simulink library "acc"  (R2021b)
settings: Solver=VariableStepAuto  StartTime=0.0  StopTime=10.0  RelTol=1e-3
undefined symbols (not defined in the file or in its folder): AACC_CondensorFanReq_X_enum, AACC_EWP1CCUReq_X_C, AACC_EWP1EDUReq_X_C, AACC_EWP1HVBReq_X_C, AACC_EWP2CCUReq_X_C, AACC_EWP2EDUReq_X_C, AACC_EWP2HVBReq_X_C, AACC_FWV1CCUReq_X_C, AACC_FWV1EDUReq_X_C, AACC_FWV1HVBReq_X_C, AACC_FWV2CCUReq_X_C, AACC_FWV2EDUReq_X_C, AACC_FWV2HVBReq_X_C, AACC_TWVCCUReq_X_C, AACC_TWVEDUReq_X_C, AACC_TWVHVBReq_X_C, ENUM_ACCMODE_CHARGING, ENUM_ACCMODE_COOLING, ENUM_ACCMODE_OFF, ENUM_ACCMODE_SERVICE, ENUM_ACREQ_COOLING, ENUM_ACREQ_NOREQUEST, ENUM_CHILLERINITREQ_NONE, ENUM_CHILLERINITREQ_START, ENUM_CHILLERINITREQ_WAITING, ENUM_CHILLERINITSTA_FINISH, ENUM_CHILLERINITSTA_INPROCESS, ENUM_COOLFANREQ_HI, ENUM_COOLFANREQ_LOW, ENUM_COOLFANREQ_OFF, ENUM_EACENDEM_SHUTDOWN, ENUM_EACENDEM_START, ENUM_EACENSTA_RUN, ENUM_EBSBRKSW_PRESSED, ENUM_EBSBRKSW_RELEASED, ENUM_EHPSENDEM_SHUTDOWN, ENUM_EHPSENDEM_START, ENUM_EPBSTARAW_SET, ENUM_GEARACTUALPOSN_N, ENUM_GEARACTUALPOSN_P, ENUM_LVBATTSTA_FAIL, ENUM_LVBATTSTA_NORMAL, ENUM_PMMMODE_CHARGE, ENUM_PMMMODE_DRIVE, ENUM_PMMMODE_LVBATCHRG, ENUM_PMMMODE_POWERUP, ENUM_POWERSTA_OFF, ENUM_POWERSTA_ON, ENUM_POWERSTA_READY, ENUM_POWERSTA_STANDBY, ENUM_PUSTATE_COMPLETED, ENUM_THCMSYS_INACTIVE, FALSE, KACC_CACEnableFailTime_s, KACC_CCUFanHighOffTemp_C, KACC_CCUFanHighOnTemp_C, KACC_CCUFanLowOffTemp_C, KACC_CCUFanLowOnTemp_C, KACC_ChillerInitTime_s, KACC_ChillerStartTime_s ... (+77)
libraries: hcu_lib x10, simulink x1
(part 1 of 2)
settings Model: Creator=13615  LastModifiedBy=zack
settings SolverCC: AlgebraicLoopSolver=TrustRegion
settings DataIOCC: SaveFormat=Array  SignalLoggingSaveFormat=ModelDataLogs  ReturnWorkspaceOutputs=off
settings OptimizationCC: BlockReduction=off  BooleanDataType=off
settings DebuggingCC: SaveWithParameterizedLinksMsg=none  UnderspecifiedInitializationDetection=Classic  MergeDetectMultiDrivingBlocksExec=none  SignalResolutionControl=TryResolveAllWithWarning  SFMachineParentedDataDiag=warning  ArithmeticOperatorsInVariantConditions=warning
settings HardwareCC: TargetUnknown=on
settings ModelReferenceCC: PropagateSignalLabelsOutOfModel=off
settings SFSimCC: CustomCodeUndefinedFunction=UseInterfaceOnly
settings ConfigComp: CovMetricSettings=dw  CovSaveCumulativeToWorkspaceVar=on  CovSaveSingleToWorkspaceVar=on

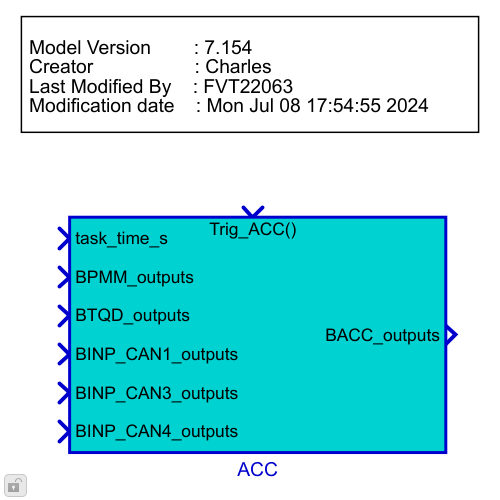
[thumbnail: Simulink's stored preview of the top-level diagram]
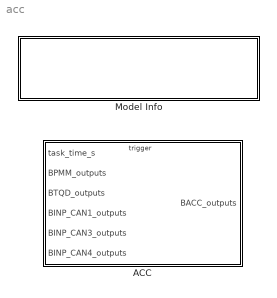
== system acc ==
  ACC : Subsystem  TreatAsAtomicUnit=on
      settings: RTWSystemCode=Nonreusable function  RTWFcnNameOpts=Use subsystem name  RTWFileNameOpts=Use subsystem name
  Model Info : Subsystem  LoadFcn=slcm LoadBlock;  InitFcn=slcm('UpdateAllCMBlocksInThisModelInit')  mask(CMBlock){InitialSaveTempField=, InitialBlockCM=None, BlockCM=None, Frame=on, SaveTempField=, DisplayStringWithTags=|, MaskDisplayString=Model Version        : 7.186\nCreator                   : Charles\nLast Modified By    : zack\nModification date    : Thu Aug 22 11:54:03 2024, HorizontalTextAlignment=Left, LeftAlignmentValue=0.02, SourceBlockDiagram=acc, TagMaxNumber=20, CMTag1=, CMTag2=, CMTag3=, CMTag4=, CMTag5=, CMTag6=, CMTag7=, CMTag8=, CMTag9=, CMTag10=, CMTag11=, CMTag12=, CMTag13=, CMTag14=, CMTag15=, CMTag16=, CMTag17=, CMTag18=, CMTag19=, CMTag20=}
      mask DisplayStringWithTags=|
      | Model Version        : %<ModelVersion>
      | Creator                   : Charles
      | Last Modified By    : %<LastModifiedBy>
      | Modification date    : %<LastModificationDate>
      mask help: This block allows revision control information to be displayed within the model.
      settings: CopyFcn=slcm CopyBlock;  DeleteFcn=slcm Cancel;  PostSaveFcn=slcm('UpdateAllCMBlocksInThisModel')  NameChangeFcn=slcm Rename;  OpenFcn=slcm
      mask Display: text(str2num(LeftAlignmentValue), 0.5, MaskDisplayString, 'HorizontalAlignment', HorizontalTextAlignment)

== system acc/ACC ==
  task_time_s : Inport
  BPMM_outputs : Inport  Port=2  OutDataTypeStr=Bus: BPMM_outputs
  BTQD_outputs : Inport  Port=3  OutDataTypeStr=Bus: BTQD_outputs
  BINP_CAN1_outputs : Inport  Port=4  OutDataTypeStr=Bus: BINP_CAN1_outputs
  BINP_CAN3_outputs : Inport  Port=5  OutDataTypeStr=Bus: BINP_CAN3_outputs
  BINP_CAN4_outputs : Inport  Port=6  OutDataTypeStr=Bus: BINP_CAN4_outputs
  Trig_ACC : TriggerPort  TriggerType=function-call  VariantControl=(inherit)
  ACC : Subsystem
  ACC1 : Subsystem  Commented=on  AncestorBlock=acc/ACC/ACC
  Bus Creator : BusCreator  Inputs=8  OutDataTypeStr=Bus: BACC_outputs  NonVirtualBus=on
  Bus Selector1 : BusSelector  OutputSignals=VINP_LVBattDet12V_V,VINP_HVBPwrAvailDchrg_kW,VINP_RrMCUDCBusVolt_V,VINP_RrMCUDCBusCurr_A
  Bus Selector2 : BusSelector  OutputSignals=VPMM_HVPwrSta_flg,VPMM_LVPwrSta_flg,VPMM_PowerSta_enum
  Bus Selector3 : BusSelector  OutputSignals=VINP_FASpeed_kph,VINP_EBSBrakeSw_enum,VINP_EACEnSta_enum,VINP_EPBParkingBrakeSta_enum
  Bus Selector4 : BusSelector  OutputSignals=VTQD_GearActualPosn_enum
  Bus Selector5 : BusSelector  OutputSignals=VINP_Z24CHAAirPressureFC2Sta_KPa,VINP_Z24CHAAirPressurePC3Sta_KPa,VINP_Z24CHAAirPressureRC1Sta_KPa
  Model Info : simulink/Model-Wide Utilities/Model Info  Frame=on  DisplayStringWithTags=|  HorizontalTextAlignment=Center  LeftAlignmentValue=0.5
      | $Id: ACC.mdl 2018-05-29 Lon $
      | Modified By %<ModifiedBy>
      | Modified Date : %<ModifiedDate>
  BACC_outputs : Outport  OutDataTypeStr=Bus: BACC_outputs  VectorParamsAs1DForOutWhenUnconnected=off
  wires:
  BPMM_outputs/1 -> Bus Selector2/1
  Bus Creator/1 -> BACC_outputs/1  "BACC_outputs"
  BINP_CAN3_outputs/1 -> Bus Selector1/1
  Bus Selector1/1 -> ACC/5(VINP_LVBattDet12V_V)  "<VINP_LVBattDet12V_V>"
  task_time_s/1 -> ACC/1(task_time_s)  "task_time_s"
  Bus Selector1/2 -> ACC/6(VINP_HVBPwrAvailDchrg_kW)  "<VINP_HVBPwrAvailDchrg_kW>"
  Bus Selector1/3 -> ACC/7(VINP_RrMCUDCBusVolt_V)  "<VINP_RrMCUDCBusVolt_V>"
  Bus Selector1/4 -> ACC/8(VINP_RrMCUDCBusCurr_A)  "<VINP_RrMCUDCBusCurr_A>"
  ACC/3(VACC_VehHVPwrAvail4THCM_W) -> Bus Creator/3
  ACC/1(VACC_HVTHCMSysAvail_enum) -> Bus Creator/1
  ACC/2(VACC_LVBattVoltSta_enum) -> Bus Creator/2
  Bus Selector2/1 -> ACC/2(VPMM_HVPwrSta_flg)  "<VPMM_HVPwrSta_flg>"
  Bus Selector2/2 -> ACC/3(VPMM_LVPwrSta_flg)  "<VPMM_LVPwrSta_flg>"
  ACC/4(VACC_EHPSEnDem_enum) -> Bus Creator/4
  ACC/5(VACC_CACPresWarnSta_flg) -> Bus Creator/5
  ACC/6(VACC_CACTempWarnSta_flg) -> Bus Creator/6
  ACC/7(VACC_EACEnDem_enum) -> Bus Creator/7
  ACC/8(VACC_EACPreSelfChkSta_flg) -> Bus Creator/8
  BINP_CAN1_outputs/1 -> Bus Selector3/1
  Bus Selector3/3 -> ACC/12(VINP_EACEnSta_enum)  "<VINP_EACEnSta_enum>"
  Bus Selector3/1 -> ACC/10(VINP_FASpeed_kph)  "<VINP_FASpeed_kph>"
  Bus Selector3/2 -> ACC/11(VINP_EBSBrakeSW_enum)  "<VINP_EBSBrakeSw_enum>"
  Bus Selector2/3 -> ACC/4(VPMM_PowerSta_enum)  "<VPMM_PowerSta_enum>"
  BTQD_outputs/1 -> Bus Selector4/1
  Bus Selector4/1 -> ACC/9(VTQD_GearActualPosn_enum)  "<VTQD_GearActualPosn_enum>"
  BINP_CAN4_outputs/1 -> Bus Selector5/1
  Bus Selector5/1 -> ACC/14(VINP_Z24CHAAirPressureFC2Sta_kPa)  "<VINP_Z24CHAAirPressureFC2Sta_KPa>"
  Bus Selector5/2 -> ACC/15(VINP_Z24CHAAirPressurePC3Sta_kPa)  "<VINP_Z24CHAAirPressurePC3Sta_KPa>"
  Bus Selector5/3 -> ACC/16(VINP_Z24CHAAirPressureRC1Sta_kPa)  "<VINP_Z24CHAAirPressureRC1Sta_KPa>"
  Bus Selector3/4 -> ACC/13(VINP_EPBParkingBrakeSta_enum)  "<VINP_EPBParkingBrakeSta_enum>"

== system acc/Model Info ==
  EmptySubsystem : Subsystem

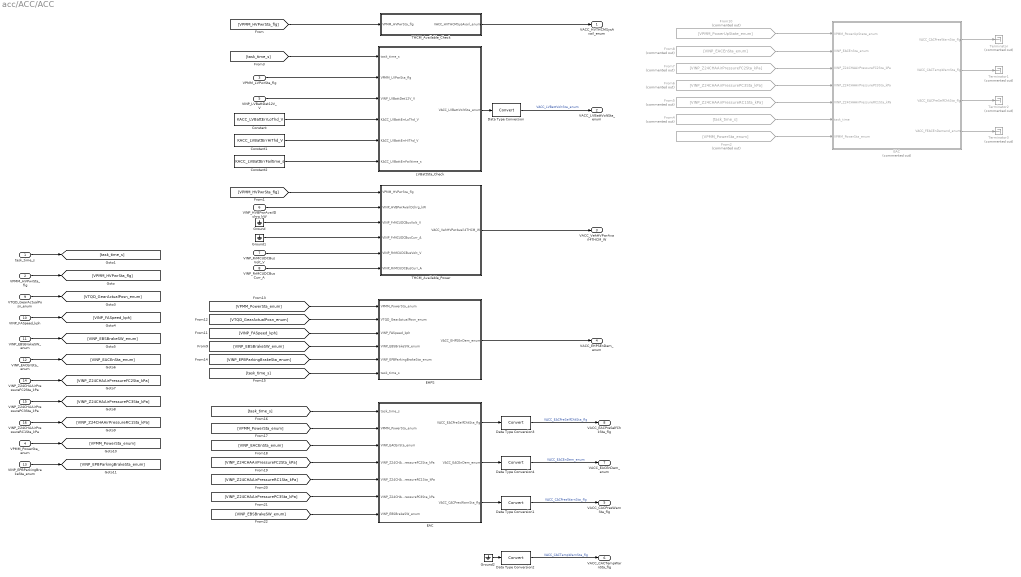
== system acc/ACC/ACC ==
  task_time_s : Inport
  VPMM_HVPwrSta_flg : Inport  Port=2
  VPMM_LVPwrSta_flg : Inport  Port=3
  VPMM_PowerSta_enum : Inport  Port=4
  VINP_LVBattDet12V_V : Inport  Port=5
  VINP_HVBPwrAvailDchrg_kW : Inport  Port=6
  VINP_RrMCUDCBusVolt_V : Inport  Port=7
  VINP_RrMCUDCBusCurr_A : Inport  Port=8
  VTQD_GearActualPosn_enum : Inport  Port=9
  VINP_FASpeed_kph : Inport  Port=10
  VINP_EBSBrakeSW_enum : Inport  Port=11
  VINP_EACEnSta_enum : Inport  Port=12
  VINP_EPBParkingBrakeSta_enum : Inport  Port=13
  VINP_Z24CHAAirPressureFC2Sta_kPa : Inport  Port=14
  VINP_Z24CHAAirPressurePC3Sta_kPa : Inport  Port=15
  VINP_Z24CHAAirPressureRC1Sta_kPa : Inport  Port=16
  Constant : Constant  Value=KACC_LVBattErrLoThd_V
  Constant1 : Constant  Value=KACC_LVBattErrHiThd_V
  Constant2 : Constant  Value=KACC_LVBattErrFailtime_s
  Data Type Conversion{,1..4} (5 alike) : DataTypeConversion
  EAC : Stateflow chart  Commented=on  TreatAsAtomicUnit=on
  "EAC " : Subsystem
  EHPS : Subsystem
  From10 : From  Commented=on  GotoTag=VPMM_PowerUpState_enum
  From2 : From  Commented=on  GotoTag=VPMM_PowerSta_enum
  From4 : From  Commented=on  GotoTag=task_time_s
  From5 : From  Commented=on  GotoTag=VINP_Z24CHAAirPressureRC1Sta_kPa
  From6 : From  Commented=on  GotoTag=VINP_Z24CHAAirPressurePC3Sta_kPa
  From7 : From  Commented=on  GotoTag=VINP_Z24CHAAirPressureFC2Sta_kPa
  From8 : From  Commented=on  GotoTag=VINP_EACEnSta_enum
  Ground : Ground
  Ground1 : Ground
  Ground2 : Ground
  LVBattSta_Check : Stateflow chart  TreatAsAtomicUnit=on
  THCM_Available_Check : Subsystem
  THCM_Available_Power : Subsystem
  Terminator{,1..3} (4 alike) : Terminator  Commented=on
  VACC_HVTHCMSysAvail_enum : Outport
  VACC_LVBattVoltSta_enum : Outport  Port=2
  VACC_VehHVPwrAvail4THCM_W : Outport  Port=3
  VACC_EHPSEnDem_enum : Outport  Port=4
  VACC_CACPresWarnSta_flg : Outport  Port=5
  VACC_CACTempWarnSta_flg : Outport  Port=6
  VACC_EACEnDem_enum : Outport  Port=7
  VACC_EACPreSelfChkSta_flg : Outport  Port=8
  wires:
  VINP_LVBattDet12V_V/1 -> LVBattSta_Check/3(VINP_LVBattDet12V_V)
  Constant/1 -> LVBattSta_Check/4(KACC_LVBattErrLoThd_V)
  Constant1/1 -> LVBattSta_Check/5(KACC_LVBattErrHiThd_V)
  Constant2/1 -> LVBattSta_Check/6(KACC_LVBattErrFailtime_s)
  LVBattSta_Check/1(VACC_LVBattVoltSta_enum) -> Data Type Conversion/1
  task_time_s/1 -> [task_time_s]
  VPMM_HVPwrSta_flg/1 -> [VPMM_HVPwrSta_flg]
  Data Type Conversion/1 -> VACC_LVBattVoltSta_enum/1  "VACC_LVBattVoltSta_enum"
  VPMM_LVPwrSta_flg/1 -> LVBattSta_Check/2(VPMM_LVPwrSta_flg)
  [VPMM_HVPwrSta_flg] -> THCM_Available_Check/1(VPMM_HVPwrSta_flg)
  THCM_Available_Check/1(VACC_HVTHCMSysAvail_enum) -> VACC_HVTHCMSysAvail_enum/1
  [VPMM_HVPwrSta_flg] -> THCM_Available_Power/1(VPMM_HVPwrSta_flg)
  THCM_Available_Power/1(VACC_VehHVPwrAvail4THCM_W) -> VACC_VehHVPwrAvail4THCM_W/1
  Ground/1 -> THCM_Available_Power/3(VINP_FrMCUDCBusVolt_V)
  Ground1/1 -> THCM_Available_Power/4(VINP_FrMCUDCBusCurr_A)
  VINP_RrMCUDCBusVolt_V/1 -> THCM_Available_Power/5(VINP_RrMCUDCBusVolt_V)
  VINP_RrMCUDCBusCurr_A/1 -> THCM_Available_Power/6(VINP_RrMCUDCBusCurr_A)
  VINP_HVBPwrAvailDchrg_kW/1 -> THCM_Available_Power/2(VINP_HVBPwrAvailDchrg_kW)
  From10/1 -> EAC/1(VPMM_PowerUpState_enum)
  From2/1 -> EAC/7(VPMM_PowerSta_enum)
  [task_time_s] -> LVBattSta_Check/1(task_time_s)
  From4/1 -> EAC/6(task_time)
  From8/1 -> EAC/2(VINP_EACEnSta_enum)
  From7/1 -> EAC/3(VINP_Z24CHAAirPressureFC2Sta_kPa)
  From6/1 -> EAC/4(VINP_Z24CHAAirPressurePC3Sta_kPa)
  From5/1 -> EAC/5(VINP_Z24CHAAirPressureRC1Sta_kPa)
  [VINP_EBSBrakeSW_enum] -> EHPS/4(VINP_EBSBrakeSW_enum)
  [VINP_FASpeed_kph] -> EHPS/3(VINP_FASpeed_kph)
  [VTQD_GearActualPosn_enum] -> EHPS/2(VTQD_GearActualPosn_enum)
  EHPS/1(VACC_EHPSEnDem_enum) -> VACC_EHPSEnDem_enum/1
  Data Type Conversion1/1 -> VACC_CACPresWarnSta_flg/1  "VACC_CACPresWarnSta_flg"
  Data Type Conversion2/1 -> VACC_CACTempWarnSta_flg/1  "VACC_CACTempWarnSta_flg"
  Data Type Conversion3/1 -> VACC_EACPreSelfChkSta_flg/1  "VACC_EACPreSelfChkSta_flg"
  Data Type Conversion4/1 -> VACC_EACEnDem_enum/1  "VACC_EACEnDem_enum"
  VTQD_GearActualPosn_enum/1 -> [VTQD_GearActualPosn_enum]
  VINP_FASpeed_kph/1 -> [VINP_FASpeed_kph]
  VINP_EBSBrakeSW_enum/1 -> [VINP_EBSBrakeSW_enum]
  VINP_EACEnSta_enum/1 -> [VINP_EACEnSta_enum]
  VINP_Z24CHAAirPressureFC2Sta_kPa/1 -> [VINP_Z24CHAAirPressureFC2Sta_kPa]
  VINP_Z24CHAAirPressurePC3Sta_kPa/1 -> [VINP_Z24CHAAirPressurePC3Sta_kPa]
  VINP_Z24CHAAirPressureRC1Sta_kPa/1 -> [VINP_Z24CHAAirPressureRC1Sta_kPa]
  VPMM_PowerSta_enum/1 -> [VPMM_PowerSta_enum]
  [VINP_EPBParkingBrakeSta_enum] -> EHPS/5(VINP_EPBParkingBrakeSta_enum)
  VINP_EPBParkingBrakeSta_enum/1 -> [VINP_EPBParkingBrakeSta_enum]
  [VPMM_PowerSta_enum] -> EHPS/1(VPMM_PowerSta_enum)
  [task_time_s] -> EHPS/6(task_time_s)
  EAC/1(VACC_CACPresWarnSta_flg) -> Terminator/1
  EAC/2(VACC_CACTempWarnSta_flg) -> Terminator1/1
  EAC/3(VACC_EACPreSelfChkSta_flg) -> Terminator2/1
  EAC/4(VACC_FEACEnDemand_enum) -> Terminator3/1
  [task_time_s] -> "EAC "/1(task_time_s)
  [VPMM_PowerSta_enum] -> "EAC "/2(VPMM_PowerSta_enum)
  [VINP_EACEnSta_enum] -> "EAC "/3(VINP_EACEnSta_enum)
  [VINP_Z24CHAAirPressureFC2Sta_kPa] -> "EAC "/4(VINP_Z24CHAAirPressureFC2Sta_kPa)
  [VINP_Z24CHAAirPressureRC1Sta_kPa] -> "EAC "/5(VINP_Z24CHAAirPressureRC1Sta_kPa)
  [VINP_Z24CHAAirPressurePC3Sta_kPa] -> "EAC "/6(VINP_Z24CHAAirPressurePC3Sta_kPa)
  [VINP_EBSBrakeSW_enum] -> "EAC "/7(VINP_EBSBrakeSW_enum)
  "EAC "/3(VACC_CACPresWarnSta_flg) -> Data Type Conversion1/1
  "EAC "/1(VACC_EACPreSelfChkSta_flg) -> Data Type Conversion3/1
  "EAC "/2(VACC_EACEnDem_enum) -> Data Type Conversion4/1
  Ground2/1 -> Data Type Conversion2/1

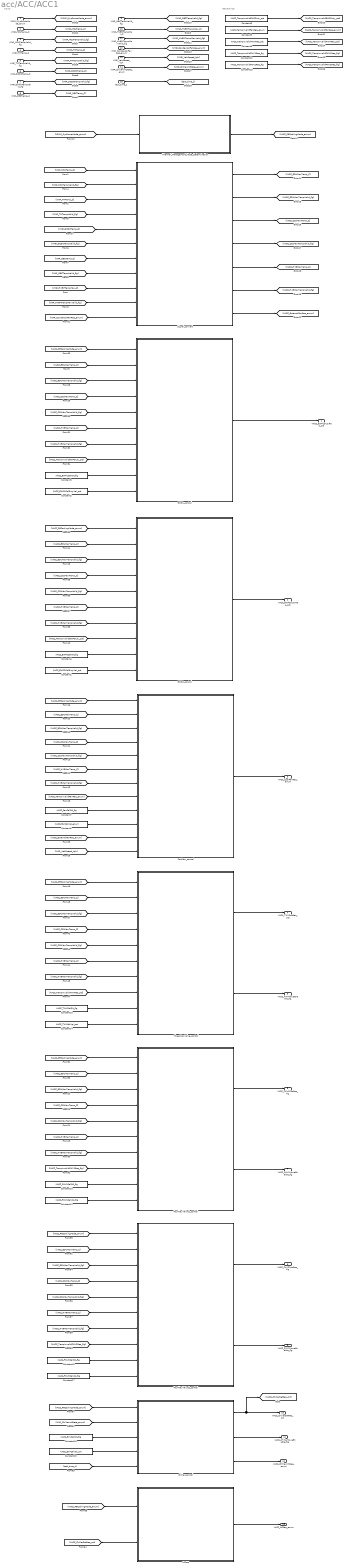
== system acc/ACC/ACC1 ==
  note: General Cal
  note: Inputs
  VPMM_SysPowerMode_enum : Inport
  VINP_MCUTemp_C : Inport  Port=2
  VINP_MCUTempValid_flg : Inport  Port=3
  VINP_TMTemp_C : Inport  Port=4
  VINP_TMTempValid_flg : Inport  Port=5
  VINP_DCDCTemp_C : Inport  Port=6
  VINP_DCDCTempValid_flg : Inport  Port=7
  VINP_OBCTemp_C : Inport  Port=8
  VINP_OBCTempValid_flg : Inport  Port=9
  VINP_HVBMTempMax_C : Inport  Port=10
  VINP_HVBMTempMaxValid_flg : Inport  Port=11
  VINP_CondensorFanReq_enum : Inport  Port=12
  VINP_VehSpeed_kph : Inport  Port=13
  VINP_ChillerInitState_enum : Inport  Port=14
  task_time_s : Inport  Port=15
  ACReq : Subsystem
  Chiller_control : Subsystem
  Constant1 : Constant  Value=KACC_EWP2CalDutyVal_pct
  Constant10 : Constant  Value=KACC_FWV1CalON_flg
  Constant11 : Constant  Value=KACC_FWV1CalVal_flg
  Constant12 : Constant  Value=KACC_TempInvalidFWV1Req_flg
  Constant13 : Constant  Value=KACC_TWVCalON_flg
  Constant14 : Constant  Value=KACC_TWVCalVal_pct
  Constant15 : Constant  Value=KACC_TempInvalidFWV2Req_flg
  Constant16 : Constant  Value=KACC_FWV2CalON_flg
  Constant17 : Constant  Value=KACC_FWV2CalVal_flg
  Constant18 : Constant  Value=KACC_EXVCalON_flg
  Constant19 : Constant  Value=KACC_EXVCalVal_cnt
  Constant2 : Constant  Value=KACC_EWP1CalDutyVal_pct
  Constant3 : Constant  Value=KACC_EWP1CalON_flg
  Constant4 : Constant  Value=KACC_EWP2CalON_flg
  Constant5 : Constant  Value=KACC_TempInvalidEWPDuty_pct
  Constant6 : Constant  Value=KACC_FanCalVal_enum
  Constant7 : Constant  Value=KACC_FanCalON_flg
  Constant8 : Constant  Value=KACC_TempInvalidTWVReq_pct
  Constant9 : Constant  Value=KACC_TempInvalidFanReq_enum
  CoolFan_control : Subsystem
  EWP1_control : Subsystem
  EWP2_control : Subsystem
  FourWayValve1_control : Subsystem
  FourWayValve2_control : Subsystem
  Signal_convert : Subsystem
  Thermal_Managemant_Mode_Determination : Subsystem
  ThreeWayValve_control : Subsystem
  VACC_EWP1DutyReq_pct : Outport  VectorParamsAs1DForOutWhenUnconnected=off
  VACC_EWP2DutyReq_pct : Outport  Port=2  VectorParamsAs1DForOutWhenUnconnected=off
  VACC_CoolFanReq_enum : Outport  Port=3  VectorParamsAs1DForOutWhenUnconnected=off
  VACC_TWVPosReq_pct : Outport  Port=4  VectorParamsAs1DForOutWhenUnconnected=off
  VACC_TWVMoveEnable_flg : Outport  Port=5  VectorParamsAs1DForOutWhenUnconnected=off
  VACC_FWV1PosReq_flg : Outport  Port=6  VectorParamsAs1DForOutWhenUnconnected=off
  VACC_FWV1MoveEnable_flg : Outport  Port=7  VectorParamsAs1DForOutWhenUnconnected=off
  VACC_FWV2PosReq_flg : Outport  Port=8  VectorParamsAs1DForOutWhenUnconnected=off
  VACC_FWV2MoveEnable_flg : Outport  Port=9  VectorParamsAs1DForOutWhenUnconnected=off
  VACC_ChillerSetReq_cnt : Outport  Port=10  VectorParamsAs1DForOutWhenUnconnected=off
  VACC_ChillerMoveEnable_flg : Outport  Port=11  VectorParamsAs1DForOutWhenUnconnected=off
  VACC_ChillerInitReq_enum : Outport  Port=12  VectorParamsAs1DForOutWhenUnconnected=off
  VACC_ACReq_enum : Outport  Port=13  VectorParamsAs1DForOutWhenUnconnected=off
  wires:
  [task_time_s] -> Chiller_control/5(task_time_s)
  task_time_s/1 -> [task_time_s]
  [VINP_ChillerInitState_enum] -> Chiller_control/2(VINP_ChillerInitState_enum)
  VINP_ChillerInitState_enum/1 -> [VINP_ChillerInitState_enum]
  Chiller_control/3(VACC_ChillerInitReq_enum) -> VACC_ChillerInitReq_enum/1  "VACC_ChillerInitReq_enum"
  Chiller_control/1(VACC_ChillerSetReq_cnt) -> [VACC_ChillerSetReq_cnt], VACC_ChillerSetReq_cnt/1  "VACC_ChillerSetReq_cnt"
  [VACC_PECoolingMode_enum] -> Chiller_control/1(VACC_PECoolingMode_enum)
  Constant18/1 -> Chiller_control/3(KACC_EXVCalON_flg)  "KACC_EXVCalON_flg"
  Constant19/1 -> Chiller_control/4(KACC_EXVCalVal_cnt)  "KACC_EXVCalVal_cnt"
  Chiller_control/2(VACC_ChillerMoveEnable_flg) -> VACC_ChillerMoveEnable_flg/1  "VACC_ChillerMoveEnable_flg"
  FourWayValve2_control/2(VACC_FWV2MoveEnable_flg) -> VACC_FWV2MoveEnable_flg/1  "VACC_FWV2MoveEnable_flg"
  Constant17/1 -> FourWayValve2_control/10(KACC_FWV2CalVal_flg)  "KACC_FWV2CalVal_flg"
  Constant16/1 -> FourWayValve2_control/9(KACC_FWV2CalON_flg)  "KACC_FWV2CalON_flg"
  [VACC_PECoolingMode_enum] -> FourWayValve2_control/1(VACC_PECoolingMode_enum)
  [VACC_CCUMaxTempValid_flg] -> FourWayValve2_control/5(VACC_CCUMaxTempValid_flg)
  [VACC_CCUMaxTemp_C] -> FourWayValve2_control/4(VACC_CCUMaxTemp_C)
  [VACC_EDUMaxTemp_C] -> FourWayValve2_control/2(VACC_EDUMaxTemp_C)
  [VACC_EDUMaxTempValid_flg] -> FourWayValve2_control/3(VACC_EDUMaxTempValid_flg)
  [VACC_HVBMaxTempValid_flg] -> FourWayValve2_control/7(VACC_HVBMaxTempValid_flg)
  FourWayValve2_control/1(VACC_FWV2PosReq_flg) -> VACC_FWV2PosReq_flg/1  "VACC_FWV2PosReq_flg"
  [VACC_HVBMaxTemp_C] -> FourWayValve2_control/6(VACC_HVBMaxTemp_C)
  [KACC_TempInvalidFWV2Req_flg] -> FourWayValve2_control/8(KACC_TempInvalidFWV2Req_flg)
  [KACC_TempInvalidFWV1Req_flg] -> FourWayValve1_control/8(KACC_TempInvalidFWV1Req_flg)
  [KACC_TempInvalidTWVReq_pct] -> ThreeWayValve_control/8(KACC_TempInvalidTWVReq_pct)
  Constant15/1 -> [KACC_TempInvalidFWV2Req_flg]  "KACC_TempInvalidFWV2Req_flg"
  Constant12/1 -> [KACC_TempInvalidFWV1Req_flg]  "KACC_TempInvalidFWV1Req_flg"
  [VACC_HVBMaxTemp_C] -> FourWayValve1_control/6(VACC_HVBMaxTemp_C)
  FourWayValve1_control/1(VACC_FWV1PosReq_flg) -> VACC_FWV1PosReq_flg/1  "VACC_FWV1PosReq_flg"
  [VACC_HVBMaxTempValid_flg] -> FourWayValve1_control/7(VACC_HVBMaxTempValid_flg)
  [VACC_EDUMaxTempValid_flg] -> FourWayValve1_control/3(VACC_EDUMaxTempValid_flg)
  [VACC_EDUMaxTemp_C] -> FourWayValve1_control/2(VACC_EDUMaxTemp_C)
  [VACC_CCUMaxTemp_C] -> FourWayValve1_control/4(VACC_CCUMaxTemp_C)
  [VACC_CCUMaxTempValid_flg] -> FourWayValve1_control/5(VACC_CCUMaxTempValid_flg)
  [VACC_PECoolingMode_enum] -> FourWayValve1_control/1(VACC_PECoolingMode_enum)
  Constant10/1 -> FourWayValve1_control/9(KACC_FWV1CalON_flg)  "KACC_FWV1CalON_flg"
  Constant11/1 -> FourWayValve1_control/10(KACC_FWV1CalVal_flg)  "KACC_FWV1CalVal_flg"
  FourWayValve1_control/2(VACC_FWV1MoveEnable_flg) -> VACC_FWV1MoveEnable_flg/1  "VACC_FWV1MoveEnable_flg"
  ThreeWayValve_control/2(VACC_TWVMoveEnable_flg) -> VACC_TWVMoveEnable_flg/1  "VACC_TWVMoveEnable_flg"
  Constant14/1 -> ThreeWayValve_control/10(KACC_TWVCalVal_pct)  "KACC_TWVCalVal_pct"
  Constant13/1 -> ThreeWayValve_control/9(KACC_TWVCalON_flg)  "KACC_TWVCalON_flg"
  Constant8/1 -> [KACC_TempInvalidTWVReq_pct]  "KACC_TempInvalidTWVReq_pct"
  [VACC_PECoolingMode_enum] -> ThreeWayValve_control/1(VACC_PECoolingMode_enum)
  [VACC_CCUMaxTempValid_flg] -> ThreeWayValve_control/5(VACC_CCUMaxTempValid_flg)
  [VACC_CCUMaxTemp_C] -> ThreeWayValve_control/4(VACC_CCUMaxTemp_C)
  [VACC_EDUMaxTemp_C] -> ThreeWayValve_control/2(VACC_EDUMaxTemp_C)
  [VACC_EDUMaxTempValid_flg] -> ThreeWayValve_control/3(VACC_EDUMaxTempValid_flg)
  [VACC_HVBMaxTempValid_flg] -> ThreeWayValve_control/7(VACC_HVBMaxTempValid_flg)
  ThreeWayValve_control/1(VACC_TWVPosReq_pct) -> VACC_TWVPosReq_pct/1  "VACC_TWVPosReq_pct"
  [VACC_HVBMaxTemp_C] -> ThreeWayValve_control/6(VACC_HVBMaxTemp_C)
  [VINP_VehSpeed_kph] -> CoolFan_control/12(VINP_VehSpeed_kph)
  VINP_VehSpeed_kph/1 -> [VINP_VehSpeed_kph]
  [VACC_ExternalFanReq_enum] -> CoolFan_control/11(VACC_ExternalFanReq_enum)
  Signal_convert/7(VACC_ExternalFanReq_enum) -> [VACC_ExternalFanReq_enum]  "VACC_ExternalFanReq_enum"
  [VINP_CondensorFanReq_enum] -> Signal_convert/11(VINP_CondensorFanReq_enum)
  [KACC_TempInvalidFanReq_enum] -> CoolFan_control/8(KACC_TempInvalidFanReq_enum)
  Constant6/1 -> CoolFan_control/10(KACC_FanCalVal_enum)  "KACC_FanCalVal_enum"
  Constant7/1 -> CoolFan_control/9(KACC_FanCalON_flg)  "KACC_FanCalON_flg"
  [VACC_CCUMaxTemp_C] -> CoolFan_control/4(VACC_CCUMaxTemp_C)
  [VACC_EDUMaxTempValid_flg] -> CoolFan_control/3(VACC_EDUMaxTempValid_flg)
  [VACC_EDUMaxTemp_C] -> CoolFan_control/2(VACC_EDUMaxTemp_C)
  [VACC_HVBMaxTempValid_flg] -> CoolFan_control/7(VACC_HVBMaxTempValid_flg)
  [VACC_HVBMaxTemp_C] -> CoolFan_control/6(VACC_HVBMaxTemp_C)
  [VACC_CCUMaxTempValid_flg] -> CoolFan_control/5(VACC_CCUMaxTempValid_flg)
  [VACC_PECoolingMode_enum] -> CoolFan_control/1(VACC_PECoolingMode_enum)
  CoolFan_control/1(VACC_CoolFanReq_enum) -> VACC_CoolFanReq_enum/1  "VACC_CoolFanReq_enum"
  EWP2_control/1(VACC_EWP2DutyReq_pct) -> VACC_EWP2DutyReq_pct/1  "VACC_EWP2DutyReq_pct"
  [VACC_PECoolingMode_enum] -> EWP2_control/1(VACC_PECoolingMode_enum)
  [VACC_CCUMaxTempValid_flg] -> EWP2_control/5(VACC_CCUMaxTempValid_flg)
  [VACC_HVBMaxTemp_C] -> EWP2_control/6(VACC_HVBMaxTemp_C)
  [VACC_HVBMaxTempValid_flg] -> EWP2_control/7(VACC_HVBMaxTempValid_flg)
  [VACC_EDUMaxTemp_C] -> EWP2_control/2(VACC_EDUMaxTemp_C)
  [VACC_EDUMaxTempValid_flg] -> EWP2_control/3(VACC_EDUMaxTempValid_flg)
  [VACC_CCUMaxTemp_C] -> EWP2_control/4(VACC_CCUMaxTemp_C)
  [KACC_TempInvalidEWPDuty_pct] -> EWP2_control/8(KACC_TempInvalidEWPDuty_pct)
  Constant4/1 -> EWP2_control/9(KACC_EWP2CalON_flg)  "KACC_EWP2CalON_flg"
  Constant1/1 -> EWP2_control/10(KACC_EWP2CalDutyVal_pct)  "KACC_EWP2CalDutyVal_pct"
  Constant2/1 -> EWP1_control/10(KACC_EWP1CalDutyVal_pct)  "KACC_EWP1CalDutyVal_pct"
  Constant3/1 -> EWP1_control/9(KACC_EWP1CalON_flg)  "KACC_EWP1CalON_flg"
  [KACC_TempInvalidEWPDuty_pct] -> EWP1_control/8(KACC_TempInvalidEWPDuty_pct)
  [VACC_CCUMaxTemp_C] -> EWP1_control/4(VACC_CCUMaxTemp_C)
  [VACC_EDUMaxTempValid_flg] -> EWP1_control/3(VACC_EDUMaxTempValid_flg)
  [VACC_EDUMaxTemp_C] -> EWP1_control/2(VACC_EDUMaxTemp_C)
  [VACC_HVBMaxTempValid_flg] -> EWP1_control/7(VACC_HVBMaxTempValid_flg)
  [VACC_HVBMaxTemp_C] -> EWP1_control/6(VACC_HVBMaxTemp_C)
  [VACC_CCUMaxTempValid_flg] -> EWP1_control/5(VACC_CCUMaxTempValid_flg)
  [VACC_PECoolingMode_enum] -> EWP1_control/1(VACC_PECoolingMode_enum)
  Constant9/1 -> [KACC_TempInvalidFanReq_enum]  "KACC_TempInvalidFanReq_enum"
  Constant5/1 -> [KACC_TempInvalidEWPDuty_pct]  "KACC_TempInvalidEWPDuty_pct"
  Signal_convert/4(VACC_CCUMaxTempValid_flg) -> [VACC_CCUMaxTempValid_flg]  "VACC_CCUMaxTempValid_flg"
  Signal_convert/5(VACC_HVBMaxTemp_C) -> [VACC_HVBMaxTemp_C]  "VACC_HVBMaxTemp_C"
  Signal_convert/3(VACC_CCUMaxTemp_C) -> [VACC_CCUMaxTemp_C]  "VACC_CCUMaxTemp_C"
  Signal_convert/6(VACC_HVBMaxTempValid_flg) -> [VACC_HVBMaxTempValid_flg]  "VACC_HVBMaxTempValid_flg"
  Signal_convert/2(VACC_EDUMaxTempValid_flg) -> [VACC_EDUMaxTempValid_flg]  "VACC_EDUMaxTempValid_flg"
  Signal_convert/1(VACC_EDUMaxTemp_C) -> [VACC_EDUMaxTemp_C]  "VACC_EDUMaxTemp_C"
  [VINP_HVBMTempMaxValid_flg] -> Signal_convert/10(VINP_HVBMTempMaxValid_flg)
  [VINP_HVBMTempMax_C] -> Signal_convert/9(VINP_HVBMTempMax_C)
  [VINP_OBCTempValid_flg] -> Signal_convert/8(VINP_OBCTempValid_flg)
  [VINP_OBCTemp_C] -> Signal_convert/7(VINP_OBCTemp_C)
  [VINP_MCUTemp_C] -> Signal_convert/1(VINP_MCUTemp_C)
  [VINP_DCDCTempValid_flg] -> Signal_convert/6(VINP_DCDCTempValid_flg)
  [VINP_MCUTempValid_flg] -> Signal_convert/2(VINP_MCUTempValid_flg)
  [VINP_TMTemp_C] -> Signal_convert/3(VINP_TMTemp_C)
  [VINP_TMTempValid_flg] -> Signal_convert/4(VINP_TMTempValid_flg)
  [VINP_DCDCTemp_C] -> Signal_convert/5(VINP_DCDCTemp_C)
  VINP_CondensorFanReq_enum/1 -> [VINP_CondensorFanReq_enum]
  VINP_DCDCTemp_C/1 -> [VINP_DCDCTemp_C]
  VINP_TMTemp_C/1 -> [VINP_TMTemp_C]
  VINP_MCUTemp_C/1 -> [VINP_MCUTemp_C]
  VPMM_SysPowerMode_enum/1 -> [VPMM_SysPowerMode_enum]
  VINP_OBCTemp_C/1 -> [VINP_OBCTemp_C]
  VINP_HVBMTempMax_C/1 -> [VINP_HVBMTempMax_C]
  VINP_MCUTempValid_flg/1 -> [VINP_MCUTempValid_flg]
  VINP_TMTempValid_flg/1 -> [VINP_TMTempValid_flg]
  VINP_DCDCTempValid_flg/1 -> [VINP_DCDCTempValid_flg]
  VINP_OBCTempValid_flg/1 -> [VINP_OBCTempValid_flg]
  VINP_HVBMTempMaxValid_flg/1 -> [VINP_HVBMTempMaxValid_flg]
  Thermal_Managemant_Mode_Determination/1(VACC_PECoolingMode_enum) -> [VACC_PECoolingMode_enum]
  [VPMM_SysPowerMode_enum] -> Thermal_Managemant_Mode_Determination/1(VPMM_SysPowerMode_enum)
  EWP1_control/1(VACC_EWP1DutyReq_pct) -> VACC_EWP1DutyReq_pct/1  "VACC_EWP1DutyReq_pct"
  [VACC_ChillerSetReq_cnt] -> ACReq/2(VACC_ChillerSetReq_cnt)
  [VACC_PECoolingMode_enum] -> ACReq/1(VACC_PECoolingMode_enum)
  ACReq/1(VACC_ACReq_enum) -> VACC_ACReq_enum/1  "VACC_ACReq_enum"

== system acc/Model Info/EmptySubsystem ==

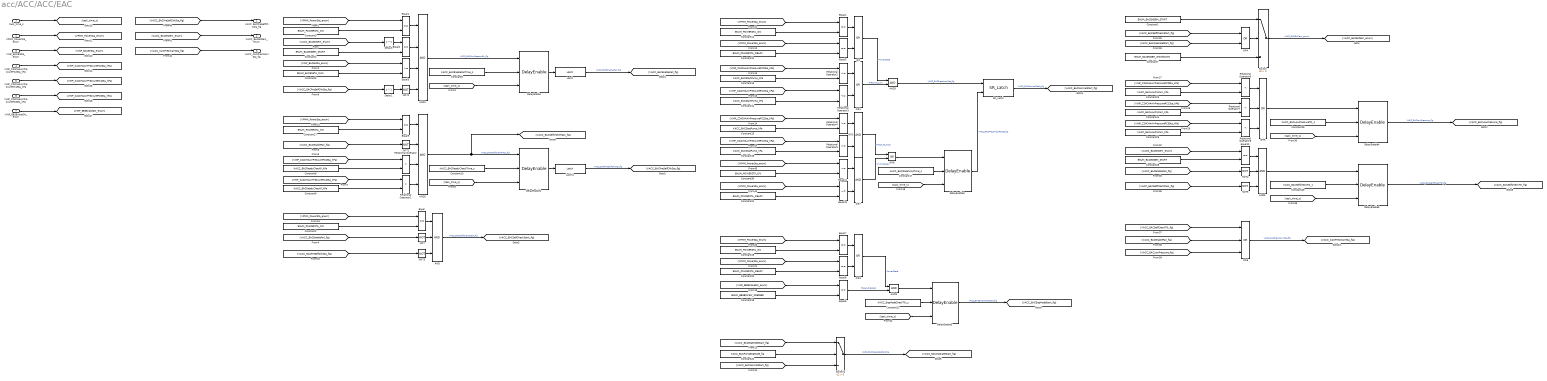
== system acc/ACC/ACC/EAC  ==
  task_time_s : Inport
  VPMM_PowerSta_enum : Inport  Port=2
  VINP_EACEnSta_enum : Inport  Port=3
  VINP_Z24CHAAirPressureFC2Sta_kPa : Inport  Port=4
  VINP_Z24CHAAirPressureRC1Sta_kPa : Inport  Port=5
  VINP_Z24CHAAirPressurePC3Sta_kPa : Inport  Port=6
  VINP_EBSBrakeSW_enum : Inport  Port=7
  AND : Logic  Inputs=3  AllPortsSameDT=off  OutDataTypeStr=boolean
  AND1 : Logic  Inputs=4  AllPortsSameDT=off  OutDataTypeStr=boolean
  AND2 : Logic  Inputs=4  AllPortsSameDT=off  OutDataTypeStr=boolean
  AND3 : Logic  AllPortsSameDT=off  OutDataTypeStr=boolean
  AND4 : Logic  AllPortsSameDT=off  OutDataTypeStr=boolean
  AND5 : Logic  Inputs=3  AllPortsSameDT=off  OutDataTypeStr=boolean
  Constant1 : Constant  Value=ENUM_EACENDEM_START
  Constant10 : Constant  Value=KACC_EACReadyCheckTime_s
  Constant{2..3,11,19,27,30} (6 alike) : Constant  Value=ENUM_POWERSTA_ON
  Constant12 : Constant  Value=ENUM_POWERSTA_READY
  Constant13 : Constant  Value=KACC_EACStartPump_kPa
  Constant14 : Constant  Value=KACC_EACStartPump_kPa
  Constant15 : Constant  Value=KACC_EACStopPump_kPa
  Constant16 : Constant  Value=KACC_EACStopPump_kPa
  Constant17 : Constant  Value=KACC_EACStopPumpTime_s
  Constant18 : Constant  Value=ENUM_EBSBRKSW_PRESSED
  Constant20 : Constant  Value=ENUM_POWERSTA_READY
  Constant21 : Constant  Value=KACC_EngModeCheckTO_s
  Constant22 : Constant  Value=KACC_EACPumpEngMode_flg
  Constant23 : Constant  Value=KACC_EACLowPrWarn_kPa
  Constant24 : Constant  Value=KACC_EACLowPrWarn_kPa
  Constant25 : Constant  Value=KACC_EACLowPrWarn_kPa
  Constant26 : Constant  Value=KACC_EACLowPressureTO_s
  Constant28 : Constant  Value=ENUM_EACENDEM_START
  Constant29 : Constant  Value=KACC_EACSelfCheckTO_s
  Constant31 : Constant  Value=ENUM_POWERSTA_READY
  Constant4 : Constant  Value=ENUM_EACENDEM_START
  Constant5 : Constant  Value=ENUM_EACENSTA_RUN
  Constant6 : Constant  Value=KACC_EACEnableFailTime_s
  Constant7 : Constant  Value=ENUM_EACENDEM_SHUTDOWN
  Constant8 : Constant  Value=KACC_EACReadyCheckP_kPa
  Constant9 : Constant  Value=KACC_EACReadyCheckP_kPa
  Delay1 : Delay  DelayLength=1
  Delay3 : Delay  DelayLength=1
  DelayEnable{,1..5} (6 alike) : hcu_lib/Basic_Blocks/DelayEnable
  Equal{,1..2,4..10} (10 alike) : RelationalOperator  Operator===  OutDataTypeStr=boolean  RndMeth=Simplest
  Equal11 : RelationalOperator  Operator=~=  OutDataTypeStr=boolean  RndMeth=Simplest
  Equal12 : RelationalOperator  Operator=~=  OutDataTypeStr=boolean  RndMeth=Simplest
  Equal3 : RelationalOperator  Operator=~=  OutDataTypeStr=boolean  RndMeth=Simplest
  Latch : hcu_lib/Basic_Blocks/Latch
  Latch1 : hcu_lib/Basic_Blocks/Latch
  NOT{,1..5} (6 alike) : Logic  Operator=NOT  AllPortsSameDT=off  OutDataTypeStr=boolean
  OR{,1,3..4,8} (5 alike) : Logic  Operator=OR  AllPortsSameDT=off  OutDataTypeStr=boolean
  OR2 : Logic  AllPortsSameDT=off  OutDataTypeStr=boolean
  OR5 : Logic  Operator=OR  Inputs=3  AllPortsSameDT=off  OutDataTypeStr=boolean
  OR6 : Logic  Operator=OR  Inputs=3  AllPortsSameDT=off  OutDataTypeStr=boolean
  OR7 : Logic  AllPortsSameDT=off  OutDataTypeStr=boolean
  Relational Operator : RelationalOperator  Operator=>  OutDataTypeStr=boolean  RndMeth=Simplest
  Relational Operator1 : RelationalOperator  Operator=>  OutDataTypeStr=boolean  RndMeth=Simplest
  Relational Operator2 : RelationalOperator  Operator=<=  OutDataTypeStr=boolean  RndMeth=Simplest
  Relational Operator3 : RelationalOperator  Operator=<=  OutDataTypeStr=boolean  RndMeth=Simplest
  Relational Operator4 : RelationalOperator  OutDataTypeStr=boolean  RndMeth=Simplest
  Relational Operator5 : RelationalOperator  OutDataTypeStr=boolean  RndMeth=Simplest
  Relational Operator6 : RelationalOperator  Operator=<  OutDataTypeStr=boolean  RndMeth=Simplest
  Relational Operator7 : RelationalOperator  Operator=<  OutDataTypeStr=boolean  RndMeth=Simplest
  Relational Operator8 : RelationalOperator  Operator=<  OutDataTypeStr=boolean  RndMeth=Simplest
  SR_Latch : hcu_lib/Basic_Blocks/SR_Latch
  Switch : Switch  Criteria=u2 > Threshold
  Switch1 : Switch  Criteria=u2 > Threshold
  VACC_EACPreSelfChkSta_flg : Outport
  VACC_EACEnDem_enum : Outport  Port=2
  VACC_CACPresWarnSta_flg : Outport  Port=3
  wires:
  VINP_EACEnSta_enum/1 -> [VINP_EACEnSta_enum]
  [VPMM_PowerSta_enum] -> Equal1/1
  [VINP_EACEnSta_enum] -> Equal3/1
  Constant5/1 -> Equal3/2
  AND/1 -> [VACC_EACSelfCheckStart_flg]  "VACC_EACSelfCheckStart_flg"
  Relational Operator4/1 -> OR2/1
  [VACC_CACPresWarnSta_flg] -> VACC_CACPresWarnSta_flg/1
  DelayEnable2/1 -> SR_Latch/2  "VACC_EACPressHighReset_flg"
  NOT2/1 -> AND1/4
  Equal/1 -> AND/1
  Constant3/1 -> Equal1/2
  [VACC_EACEnableFail_flg] -> NOT1/1
  Constant21/1 -> DelayEnable3/2
  Constant1/1 -> Switch/1
  SR_Latch/1 -> [VACC_EACNormalStart_flg]  "VACC_EACNormalStart_flg"
  VINP_EBSBrakeSW_enum/1 -> [VINP_EBSBrakeSW_enum]
  Equal8/1 -> OR3/2
  [VPMM_PowerSta_enum] -> Equal4/1
  Constant9/1 -> Relational Operator1/2
  Equal1/1 -> AND1/1
  [VINP_Z24CHAAirPressureFC2Sta_kPa] -> Relational Operator/1
  Constant11/1 -> Equal4/2
  [VPMM_PowerSta_enum] -> Equal9/1
  Equal2/1 -> AND1/2
  AND3/1 -> SR_Latch/1  "VACC_EACPressLowSet_flg"
  [VACC_EACEnableFail_flg] -> NOT/1
  Delay1/1 -> NOT2/1
  Constant15/1 -> Relational Operator4/2
  AND2/1 -> [VACC_EACSelfCheckPass_flg], DelayEnable1/1  "VACC_EACSelfCheckPass_flg"
  [VACC_EACLowPressure_flg] -> OR6/3
  NOT3/1 -> AND/3
  Relational Operator2/1 -> OR1/1
  DelayEnable/1 -> Latch/1
  [task_time_s] -> DelayEnable1/3
  [task_time_s] -> DelayEnable3/3
  Constant8/1 -> Relational Operator/2
  VINP_Z24CHAAirPressureRC1Sta_kPa/1 -> [VINP_Z24CHAAirPressureRC1Sta_kPa]
  DelayEnable1/1 -> Latch1/1
  [VACC_EACPreSelfChkSta_flg] -> NOT3/1
  OR/1 -> AND3/1  "PowerState"
  DelayEnable3/1 -> [VACC_EACEngModeStart_flg]  "VACC_EACEngModeStart_flg"
  Latch1/1 -> [VACC_EACPreSelfChkSta_flg]  "VACC_EACPreSelfChkSta_flg"
  [VACC_EACPreSelfChkSta_flg] -> Delay1/1
  [VPMM_PowerSta_enum] -> Equal/1
  Constant18/1 -> Equal6/2
  Constant10/1 -> DelayEnable1/2
  Constant6/1 -> DelayEnable/2
  Constant4/1 -> Equal2/2
  Equal4/1 -> OR/1
  [VINP_Z24CHAAirPressureRC1Sta_kPa] -> Relational Operator5/1
  Constant12/1 -> Equal5/2
  Constant13/1 -> Relational Operator2/2
  Equal5/1 -> OR/2
  [VACC_EACEnableFail_flg] -> OR6/2
  [VPMM_PowerSta_enum] -> Equal8/1
  [VPMM_PowerSta_enum] -> Equal5/1
  Relational Operator5/1 -> OR2/2
  Constant17/1 -> DelayEnable2/2
  Constant22/1 -> Switch1/2
  [VINP_Z24CHAAirPressureFC2Sta_kPa] -> Relational Operator2/1
  [VINP_EBSBrakeSW_enum] -> Equal6/1
  [VINP_Z24CHAAirPressureFC2Sta_kPa] -> Relational Operator4/1
  Latch/1 -> [VACC_EACEnableFail_flg]  "VACC_EACEnableFail_flg"
  [VPMM_PowerSta_enum] -> Equal7/1
  Constant19/1 -> Equal7/2
  Constant20/1 -> Equal8/2
  Constant24/1 -> Relational Operator7/2
  [VINP_Z24CHAAirPressureRC1Sta_kPa] -> Relational Operator1/1
  Equal6/1 -> AND4/2  "Break_Pressed"
  AND4/1 -> DelayEnable3/1
  OR3/1 -> AND4/1  "PowerState"
  VINP_Z24CHAAirPressureFC2Sta_kPa/1 -> [VINP_Z24CHAAirPressureFC2Sta_kPa]
  Constant7/1 -> Switch/3
  Switch/1 -> [VACC_EACEnDem_enum]  "VACC_EACEnDem_enum"
  task_time_s/1 -> [task_time_s]
  OR6/1 -> [VACC_CACPresWarnSta_flg]  "VACC_CACPresWarnSta_flg"
  [VACC_EACNormalStart_flg] -> Switch1/3
  [VACC_EACEnDem_enum] -> VACC_EACEnDem_enum/1
  VINP_Z24CHAAirPressurePC3Sta_kPa/1 -> [VINP_Z24CHAAirPressurePC3Sta_kPa]
  [VACC_EACPreSelfChkSta_flg] -> VACC_EACPreSelfChkSta_flg/1
  Constant25/1 -> Relational Operator8/2
  Constant26/1 -> DelayEnable4/2
  [VINP_Z24CHAAirPressureRC1Sta_kPa] -> Relational Operator7/1
  [VINP_Z24CHAAirPressurePC3Sta_kPa] -> Relational Operator8/1
  [VINP_Z24CHAAirPressureFC2Sta_kPa] -> Relational Operator6/1
  OR4/1 -> Switch/2
  OR1/1 -> AND3/2  "Pressure_Low"
  NOT/1 -> AND/2
  OR5/1 -> DelayEnable4/1
  [VACC_EACOperateStart_flg] -> OR4/2
  [VACC_EACSelfCheckStart_flg] -> OR4/1
  [VACC_EACEnDem_enum] -> Equal10/1
  [task_time_s] -> DelayEnable/3
  Relational Operator1/1 -> AND2/4
  Relational Operator/1 -> AND2/3
  Constant14/1 -> Relational Operator3/2
  NOT1/1 -> AND2/2
  NOT4/1 -> AND5/2
  AND5/1 -> DelayEnable5/1
  Equal10/1 -> AND5/1
  Relational Operator7/1 -> OR5/2
  Constant23/1 -> Relational Operator6/2
  Constant28/1 -> Equal10/2
  DelayEnable4/1 -> [VACC_EACLowPressure_flg]  "VACC_EACLowPressure_flg"
  Equal3/1 -> AND1/3
  Relational Operator8/1 -> OR5/3
  [VINP_Z24CHAAirPressureRC1Sta_kPa] -> Relational Operator3/1
  [VACC_EACEngModeStart_flg] -> Switch1/1
  Constant2/1 -> Equal/2
  Relational Operator6/1 -> OR5/1
  Constant16/1 -> Relational Operator5/2
  [task_time_s] -> DelayEnable4/3
  Switch1/1 -> [VACC_EACOperateStart_flg]  "VACC_EACOperateStart_flg"
  Equal7/1 -> OR3/1
  Relational Operator3/1 -> OR1/2
  AND1/1 -> DelayEnable/1  "VACC_EACRunResponErr_flg"
  Equal9/1 -> AND2/1
  Constant27/1 -> Equal9/2
  [task_time_s] -> DelayEnable2/3
  NOT5/1 -> AND5/3
  VPMM_PowerSta_enum/1 -> [VPMM_PowerSta_enum]
  [VACC_EACSelfCheckTO_flg] -> OR6/1
  [task_time_s] -> DelayEnable5/3
  Constant29/1 -> DelayEnable5/2
  [VACC_EACEnDem_enum] -> Delay3/1
  Delay3/1 -> Equal2/1
  [VACC_EACSelfCheckPass_flg] -> NOT5/1
  [VACC_EACEnableFail_flg] -> NOT4/1
  DelayEnable5/1 -> [VACC_EACSelfCheckTO_flg]  "VACC_EACSelfCheckTO_flg"
  Equal11/1 -> OR7/1
  [VPMM_PowerSta_enum] -> Equal12/1
  Constant30/1 -> Equal11/2
  Equal12/1 -> OR7/2
  [VPMM_PowerSta_enum] -> Equal11/1
  Constant31/1 -> Equal12/2
  OR8/1 -> DelayEnable2/1
  OR2/1 -> OR8/1  "Pressure_High"
  OR7/1 -> OR8/2  "!= On/Ready"

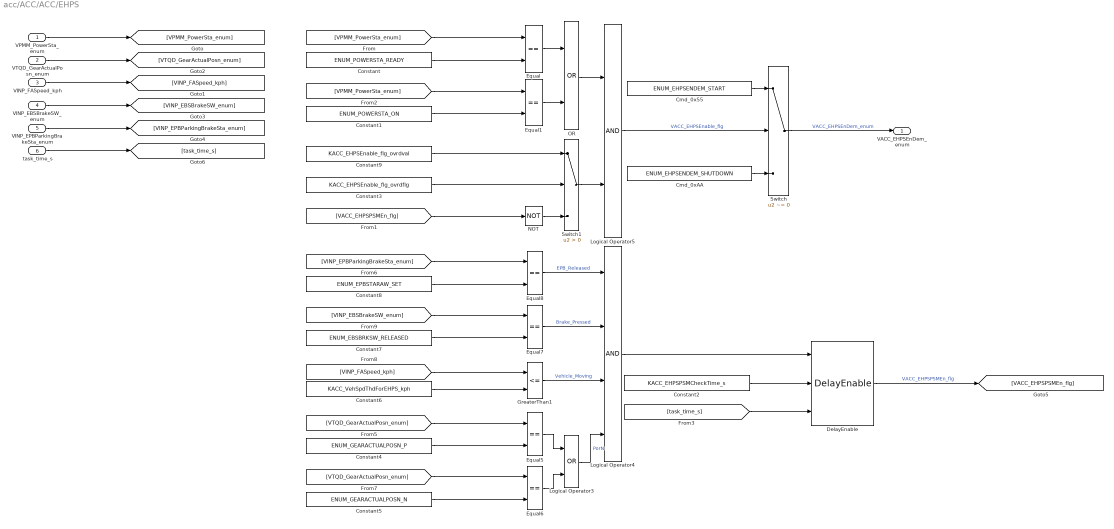
== system acc/ACC/ACC/EHPS ==
  VPMM_PowerSta_enum : Inport
  VTQD_GearActualPosn_enum : Inport  Port=2
  VINP_FASpeed_kph : Inport  Port=3
  VINP_EBSBrakeSW_enum : Inport  Port=4
  VINP_EPBParkingBrakeSta_enum : Inport  Port=5
  task_time_s : Inport  Port=6
  Cmd_0x55 : Constant  Value=ENUM_EHPSENDEM_START
  Cmd_0xAA : Constant  Value=ENUM_EHPSENDEM_SHUTDOWN
  Constant : Constant  Value=ENUM_POWERSTA_READY
  Constant1 : Constant  Value=ENUM_POWERSTA_ON
  Constant2 : Constant  Value=KACC_EHPSPSMCheckTime_s
  Constant3 : Constant  Value=KACC_EHPSEnable_flg_ovrdflg
  Constant4 : Constant  Value=ENUM_GEARACTUALPOSN_P
  Constant5 : Constant  Value=ENUM_GEARACTUALPOSN_N
  Constant6 : Constant  Value=KACC_VehSpdThdForEHPS_kph
  Constant7 : Constant  Value=ENUM_EBSBRKSW_RELEASED  OutDataTypeStr=Inherit: Inherit via back propagation
  Constant8 : Constant  Value=ENUM_EPBSTARAW_SET
  Constant9 : Constant  Value=KACC_EHPSEnable_flg_ovrdval
  DelayEnable : hcu_lib/Basic_Blocks/DelayEnable
  Equal{,1,5..8} (6 alike) : RelationalOperator  Operator===  OutDataTypeStr=boolean  RndMeth=Simplest
  GreaterThan1 : RelationalOperator  Operator=<=  OutDataTypeStr=boolean  RndMeth=Simplest
  Logical Operator3 : Logic  Operator=OR  AllPortsSameDT=off  OutDataTypeStr=boolean
  Logical Operator4 : Logic  Inputs=4  AllPortsSameDT=off  OutDataTypeStr=boolean
  Logical Operator5 : Logic  AllPortsSameDT=off  OutDataTypeStr=boolean
  NOT : Logic  Operator=NOT  AllPortsSameDT=off  OutDataTypeStr=boolean
  OR : Logic  Operator=OR  AllPortsSameDT=off  OutDataTypeStr=boolean
  Switch : Switch  Criteria=u2 ~= 0
      settings: AttributesFormatString=%<Criteria>
  Switch1 : Switch  Criteria=u2 > Threshold
  VACC_EHPSEnDem_enum : Outport
  wires:
  VPMM_PowerSta_enum/1 -> [VPMM_PowerSta_enum]
  Constant/1 -> Equal/2
  VTQD_GearActualPosn_enum/1 -> [VTQD_GearActualPosn_enum]
  VINP_FASpeed_kph/1 -> [VINP_FASpeed_kph]
  VINP_EBSBrakeSW_enum/1 -> [VINP_EBSBrakeSW_enum]
  [VTQD_GearActualPosn_enum] -> Equal5/1
  Constant4/1 -> Equal5/2
  [VINP_FASpeed_kph] -> GreaterThan1/1
  Equal6/1 -> Logical Operator3/2
  [VINP_EBSBrakeSW_enum] -> Equal7/1
  Equal7/1 -> Logical Operator4/2  "Brake_Pressed"
  Equal8/1 -> Logical Operator4/1  "EPB_Released"
  Constant7/1 -> Equal7/2
  GreaterThan1/1 -> Logical Operator4/3  "Vehicle_Moving"
  Equal5/1 -> Logical Operator3/1
  Logical Operator3/1 -> Logical Operator4/4  "PorN"
  Constant5/1 -> Equal6/2
  [VTQD_GearActualPosn_enum] -> Equal6/1
  Constant8/1 -> Equal8/2
  [VINP_EPBParkingBrakeSta_enum] -> Equal8/1
  Constant6/1 -> GreaterThan1/2
  Switch/1 -> VACC_EHPSEnDem_enum/1  "VACC_EHPSEnDem_enum"
  Cmd_0x55/1 -> Switch/1
  Cmd_0xAA/1 -> Switch/3
  VINP_EPBParkingBrakeSta_enum/1 -> [VINP_EPBParkingBrakeSta_enum]
  Logical Operator5/1 -> Switch/2  "VACC_EHPSEnable_flg"
  [VPMM_PowerSta_enum] -> Equal/1
  [VPMM_PowerSta_enum] -> Equal1/1
  Constant1/1 -> Equal1/2
  OR/1 -> Logical Operator5/1
  Equal1/1 -> OR/2
  Equal/1 -> OR/1
  task_time_s/1 -> [task_time_s]
  [task_time_s] -> DelayEnable/3
  Constant2/1 -> DelayEnable/2
  Logical Operator4/1 -> DelayEnable/1
  DelayEnable/1 -> [VACC_EHPSPSMEn_flg]  "VACC_EHPSPSMEn_flg"
  Switch1/1 -> Logical Operator5/2
  NOT/1 -> Switch1/3
  [VACC_EHPSPSMEn_flg] -> NOT/1
  Constant9/1 -> Switch1/1
  Constant3/1 -> Switch1/2

== system acc/ACC/ACC/THCM_Available_Check ==
  VPMM_HVPwrSta_flg : Inport
  Constant4 : Constant  Value=ENUM_THCMSYS_INACTIVE
  Constant5 : Constant  Value=KACC_HVTHCMSysAvail_enum_ovrdflg
  Constant6 : Constant  Value=KACC_HVTHCMSysAvail_enum_ovrdval
  Constant7 : Constant  Value=ENUM_THCMSYS_INACTIVE
  Switch2 : Switch  Criteria=u2 ~= 0
      settings: AttributesFormatString=<%<Criteria>>
  Switch3 : Switch  Criteria=u2 ~= 0
      settings: AttributesFormatString=<%<Criteria>>
  VACC_HVTHCMSysAvail_enum : Outport
  wires:
  Constant5/1 -> Switch3/2
  Constant4/1 -> Switch2/3
  Switch2/1 -> VACC_HVTHCMSysAvail_enum/1  "VACC_HVTHCMSysAvail_enum"
  Switch3/1 -> Switch2/1
  VPMM_HVPwrSta_flg/1 -> Switch2/2
  Constant6/1 -> Switch3/1
  Constant7/1 -> Switch3/3

== system acc/ACC/ACC/THCM_Available_Power ==
  VPMM_HVPwrSta_flg : Inport
  VINP_HVBPwrAvailDchrg_kW : Inport  Port=2
  VINP_FrMCUDCBusVolt_V : Inport  Port=3
  VINP_FrMCUDCBusCurr_A : Inport  Port=4
  VINP_RrMCUDCBusVolt_V : Inport  Port=5
  VINP_RrMCUDCBusCurr_A : Inport  Port=6
  Add : Sum
  Add1 : Sum  Inputs=+-
  Constant10 : Constant  Value=KACC_HVPwrAvail4THCM_W_ovrdval
  Constant8 : Constant  Value=ZERO_FLOAT
  Constant9 : Constant  Value=KACC_HVPwrAvail4THCM_W_ovrdflg
  Product : Product
  Product1 : Product
  Saturation : Saturate  UpperLimit=KACC_THCMMaxPwrAvail_W  LowerLimit=0
      settings: AttributesFormatString=|
      | Upper Limit: %<UpperLimit>
      | Lower Limit: %<LowerLimit>
  Switch1 : Switch  Criteria=u2 ~= 0
      settings: AttributesFormatString=<%<Criteria>>
  Switch4 : Switch  Criteria=u2 ~= 0
      settings: AttributesFormatString=<%<Criteria>>
  VACC_VehHVPwrAvail4THCM_W : Outport
  wires:
  Constant10/1 -> Switch4/1
  Switch4/1 -> Switch1/1
  Saturation/1 -> Switch4/3
  Constant8/1 -> Switch1/3
  VPMM_HVPwrSta_flg/1 -> Switch1/2
  Switch1/1 -> VACC_VehHVPwrAvail4THCM_W/1  "VACC_VehHVPwrAvail4THCM_W"
  Constant9/1 -> Switch4/2
  VINP_RrMCUDCBusCurr_A/1 -> Product/2
  VINP_RrMCUDCBusVolt_V/1 -> Product/1
  VINP_FrMCUDCBusCurr_A/1 -> Product1/2
  VINP_FrMCUDCBusVolt_V/1 -> Product1/1
  Product1/1 -> Add/1
  Product/1 -> Add/2
  VINP_HVBPwrAvailDchrg_kW/1 -> Add1/1
  Add/1 -> Add1/2
  Add1/1 -> Saturation/1

== system acc/ACC/ACC1/ACReq ==
  VACC_PECoolingMode_enum : Inport
  VACC_ChillerSetReq_cnt : Inport  Port=2
  Constant1 : Constant  Value=ZERO_INT
  Constant10 : Constant  Value=ENUM_ACCMODE_CHARGING
  Constant11 : Constant  Value=ENUM_ACCMODE_COOLING
  Constant2 : Constant  Value=ENUM_ACREQ_COOLING
  Constant3 : Constant  Value=ENUM_ACREQ_NOREQUEST
  OR2 : Logic  Operator=OR  AllPortsSameDT=off  OutDataTypeStr=boolean
  OR3 : Logic  AllPortsSameDT=off  OutDataTypeStr=boolean
  Relational Operator1 : RelationalOperator  Operator===  OutDataTypeStr=boolean  RndMeth=Simplest
  Relational Operator2 : RelationalOperator  Operator=>  OutDataTypeStr=boolean  RndMeth=Simplest
  Relational Operator3 : RelationalOperator  Operator===  OutDataTypeStr=boolean  RndMeth=Simplest
  Switch2 : Switch  Criteria=u2 ~= 0
      settings: AttributesFormatString=%<Criteria>
  VACC_ACReq_enum : Outport
  wires:
  VACC_ChillerSetReq_cnt/1 -> [VACC_ChillerSetReq_cnt]
  VACC_PECoolingMode_enum/1 -> [VACC_PECoolingMode_enum]
  OR2/1 -> OR3/1
  [VACC_PECoolingMode_enum] -> Relational Operator1/1
  [VACC_PECoolingMode_enum] -> Relational Operator3/1
  Constant11/1 -> Relational Operator3/2
  Constant10/1 -> Relational Operator1/2
  Relational Operator3/1 -> OR2/1
  Relational Operator1/1 -> OR2/2
  OR3/1 -> Switch2/2
  [VACC_ChillerSetReq_cnt] -> Relational Operator2/1
  Constant1/1 -> Relational Operator2/2
  Relational Operator2/1 -> OR3/2
  Switch2/1 -> VACC_ACReq_enum/1
  Constant2/1 -> Switch2/1
  Constant3/1 -> Switch2/3

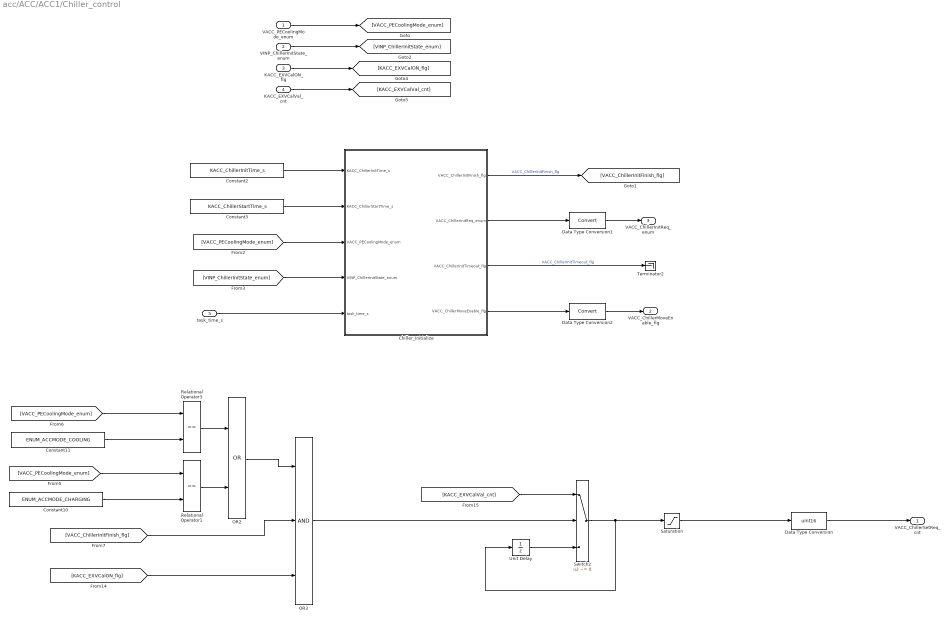
== system acc/ACC/ACC1/Chiller_control ==
  VACC_PECoolingMode_enum : Inport
  VINP_ChillerInitState_enum : Inport  Port=2
  KACC_EXVCalON_flg : Inport  Port=3
  KACC_EXVCalVal_cnt : Inport  Port=4
  task_time_s : Inport  Port=5
  Chiller_Initialize : Stateflow chart  TreatAsAtomicUnit=on
  Constant10 : Constant  Value=ENUM_ACCMODE_CHARGING
  Constant11 : Constant  Value=ENUM_ACCMODE_COOLING
  Constant2 : Constant  Value=KACC_ChillerInitTime_s
  Constant3 : Constant  Value=KACC_ChillerStartTime_s
  Data Type Conversion : DataTypeConversion  OutDataTypeStr=uint16
  Data Type Conversion1 : DataTypeConversion
  Data Type Conversion2 : DataTypeConversion
  OR2 : Logic  Operator=OR  AllPortsSameDT=off  OutDataTypeStr=boolean
  OR3 : Logic  Inputs=3  AllPortsSameDT=off  OutDataTypeStr=boolean
  Relational Operator1 : RelationalOperator  Operator===  OutDataTypeStr=boolean  RndMeth=Simplest
  Relational Operator3 : RelationalOperator  Operator===  OutDataTypeStr=boolean  RndMeth=Simplest
  Saturation : Saturate  UpperLimit=576  LowerLimit=0
      settings: AttributesFormatString=|
      | LowerLimi: %<LowerLimit>
      | UpperLimit: %<UpperLimit>
  Switch2 : Switch  Criteria=u2 ~= 0
      settings: AttributesFormatString=%<Criteria>
  Terminator2 : Terminator
  Unit Delay : UnitDelay  SampleTime=-1  HasFrameUpgradeWarning=on
      settings: AttributesFormatString=InitialCondition: %<InitialCondition>
  VACC_ChillerSetReq_cnt : Outport
  VACC_ChillerMoveEnable_flg : Outport  Port=2
  VACC_ChillerInitReq_enum : Outport  Port=3
  wires:
  Chiller_Initialize/4(VACC_ChillerMoveEnable_flg) -> Data Type Conversion2/1
  Data Type Conversion2/1 -> VACC_ChillerMoveEnable_flg/1
  Data Type Conversion1/1 -> VACC_ChillerInitReq_enum/1
  Switch2/1 -> Saturation/1, Unit Delay/1
  Unit Delay/1 -> Switch2/3
  Saturation/1 -> Data Type Conversion/1
  OR3/1 -> Switch2/2
  [KACC_EXVCalON_flg] -> OR3/3
  Chiller_Initialize/3(VACC_ChillerInitTimeout_flg) -> Terminator2/1  "VACC_ChillerInitTimeout_flg"
  Chiller_Initialize/2(VACC_ChillerInitReq_enum) -> Data Type Conversion1/1
  Relational Operator1/1 -> OR2/2
  Relational Operator3/1 -> OR2/1
  Constant10/1 -> Relational Operator1/2
  Constant11/1 -> Relational Operator3/2
  [VACC_PECoolingMode_enum] -> Relational Operator3/1
  [VACC_PECoolingMode_enum] -> Relational Operator1/1
  OR2/1 -> OR3/1
  [VACC_ChillerInitFinish_flg] -> OR3/2
  Data Type Conversion/1 -> VACC_ChillerSetReq_cnt/1
  task_time_s/1 -> Chiller_Initialize/5(task_time_s)
  [VACC_PECoolingMode_enum] -> Chiller_Initialize/3(VACC_PECoolingMode_enum)
  [VINP_ChillerInitState_enum] -> Chiller_Initialize/4(VINP_ChillerInitState_enum)
  Constant3/1 -> Chiller_Initialize/2(KACC_ChillerStartTime_s)
  Constant2/1 -> Chiller_Initialize/1(KACC_ChillerInitTime_s)
  Chiller_Initialize/1(VACC_ChillerInitFinish_flg) -> [VACC_ChillerInitFinish_flg]  "VACC_ChillerInitFinish_flg"
  [KACC_EXVCalVal_cnt] -> Switch2/1
  KACC_EXVCalVal_cnt/1 -> [KACC_EXVCalVal_cnt]
  KACC_EXVCalON_flg/1 -> [KACC_EXVCalON_flg]
  VACC_PECoolingMode_enum/1 -> [VACC_PECoolingMode_enum]
  VINP_ChillerInitState_enum/1 -> [VINP_ChillerInitState_enum]
